simulink model "HybridInverter"  (R2024b)
settings: Solver=ode23t  StartTime=0.0  StopTime=1  RelTol=1e-3
undefined symbols (not defined in the file): Ion, Lithium
libraries: spsCurrentMeasurementLib x8, spsSeriesRLCBranchLib x8, spsVoltageMeasurementLib x8, spsIGBTDiodeLib x7, spsIdealSwitchLib x5, slpidlib x3, spsSeriesRLCLoadLib x3, spsFirstOrderFilterLib x2, simulink x2, spsACVoltageSourceLib x1, spsAlphaBetaZerotodq0Lib x1, spsBatteryLib x1
settings Model: SimulationMode=accelerator  Creator=USER  LastModifiedBy=USER

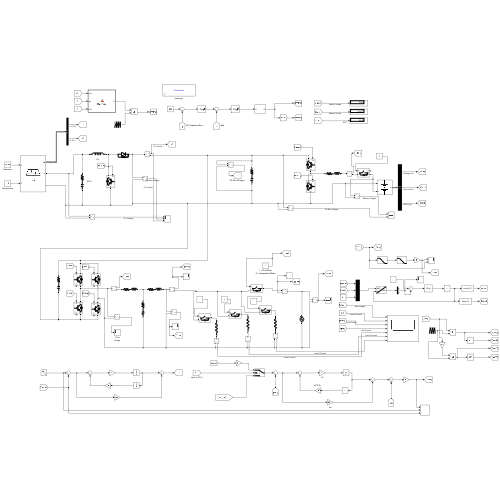
[thumbnail: Simulink's stored preview of the top-level diagram]
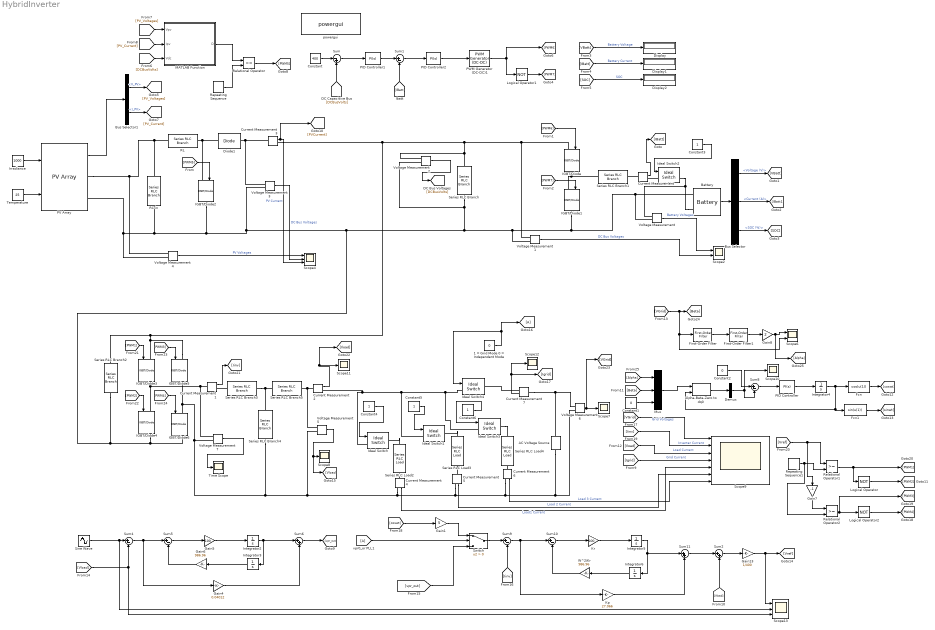
== system HybridInverter ==
  1 = Grid Mode 0 = Independent Mode : Constant  Value=0
  AC Voltage Source : spsACVoltageSourceLib/AC Voltage Source  Amplitude=325  Phase=0  Frequency=50  SampleTime=0  Measurements=None  BusType=swing  Pref=10e3  Qref=0  Qmin=-inf  Qmax=+inf
  Alpha-Beta-Zero to dq0 : spsAlphaBetaZerotodq0Lib/Alpha-Beta-Zero to dq0  Alignment=90 degrees behind phase A axis
  Battery : spsBatteryLib/Battery  BatType=Lithium-Ion  NomV=200  NomQ=15  SOC=55  Batt_Tr=1  PresetModel=on  MaxQ=15  MinV=150  FullV=232.7974  Dis_rate=6.5217  R=0.13333  Normal_OP=13.5652  expZone="[216.0772     0.7369565]"
  Bus Selector : BusSelector  OutputSignals=Voltage (V),Current (A),SOC (%)
  Bus Selector1 : BusSelector  OutputSignals=V_PV,I_PV
  Constant : Constant  Value=400
  Constant1 : Constant  Value=0
  Constant2 : Constant  Value=0
  Constant{3..6} (4 alike) : Constant
  Current Measurement{,1..7} (8 alike) : spsCurrentMeasurementLib/Current Measurement  PhasorSimulation=off  OutputType=Complex  PSBequivalent=0
  Demux : Demux  Outputs=3
  Diode1 : spsDiodeLib/Diode  Ron=0.001  Lon=0  Vf=0.8  IC=0  UseSnubber=0  Rs=500  Cs=250e-9  Measurements=off
  Display : Display
  Display1 : Display
  Display2 : Display
  Fcn : Fcn  Expr=cos(u(1))
  Fcn1 : Fcn  Expr=sin(u(1))
  First-Order Filter : spsFirstOrderFilterLib/First-Order Filter  FilterType=Lowpass  Tc=1/(2*pi*50)  Ts=0  Initialize=off  Vac_Init=[0, 0, 60]  Vdc_Init=0  PlotResponse=off  FreqRange="[0,  200,  1]"
  First-Order Filter1 : spsFirstOrderFilterLib/First-Order Filter  FilterType=Lowpass  Tc=1/(2*pi*50)  Ts=0  Initialize=off  Vac_Init=[0, 0, 60]  Vdc_Init=0  PlotResponse=off  FreqRange="[0,  200,  1]"
  Gain1 : Gain  Gain=5
  Gain13 : Gain  Gain=1/400
  Gain4 : Gain  Gain=0.04012
  Gain5 : Gain  Gain=100
  Gain6 : Gain  Gain=986.96
  Gain7 : Gain  Gain=-1
  Gain8 : Gain  Gain=2
  Goto16 : Goto
  IGBT/Diode : spsIGBTDiodeLib/IGBT//Diode  Ron=1e-3  Rs=1e5  Cs=inf  Measurements=off
  IGBT/Diode1 : spsIGBTDiodeLib/IGBT//Diode  Ron=1e-3  Rs=1e5  Cs=inf  Measurements=off
  IGBT/Diode2 : spsIGBTDiodeLib/IGBT//Diode  Ron=1e-3  Rs=1e5  Cs=inf  Measurements=off
  IGBT/Diode{3..6} (4 alike) : spsIGBTDiodeLib/IGBT//Diode  Ron=1e-3  Rs=1e5  Cs=inf  Measurements=on
  Ideal Switch{,1,3..4} (4 alike) : spsIdealSwitchLib/Ideal Switch  Ron=0.001  Lon=0  IC=0  Rs=1e5  Cs=inf  Measurements=off
  Ideal Switch2 : spsIdealSwitchLib/Ideal Switch  Ron=0.001  Lon=0  IC=0  Rs=1e5  Cs=inf  Measurements=on
  Integrator{2..6} (5 alike) : Integrator
  Irradiance : Constant  Value=1000
  Kp : Gain  Gain=27.066
  Kr : Gain  Gain=100
  Logical Operator : Logic  Operator=NOT  AllPortsSameDT=off  OutDataTypeStr=boolean
  Logical Operator1 : Logic  Operator=NOT  AllPortsSameDT=off  OutDataTypeStr=boolean
  Logical Operator2 : Logic  Operator=NOT  AllPortsSameDT=off  OutDataTypeStr=boolean
  MATLAB Function : MATLAB Function  TreatAsAtomicUnit=on
  Mux : Mux  Inputs=3
  PID Controller : slpidlib/PID Controller  Controller=PI  Form=Parallel  TimeDomain=Continuous-time  UseExternalTs=off  SampleTime=-1  IntegratorMethod=Forward Euler  FilterMethod=Forward Euler  ControllerParametersSource=internal  P=10  I=50000  UseKiTs=off  D=0  UseExternalDerivativeSource=off  N=100  UseFilter=on  TunerSelectOption=Transfer Function Based (PID Tuner App)  InitialConditionSource=internal  InitialConditionForIntegrator=0  InitialConditionForFilter=0  DifferentiatorICPrevScaledInput=0  ExternalReset=none  TrackingMode=off  Kt=1  LimitOutput=off  SatLimitsSource=internal  UpperSaturationLimit=inf  LowerSaturationLimit=-inf  LinearizeAsGain=on  AntiWindupMode=none  Kb=1  LimitIntegrator=off  UpperIntegratorSaturationLimit=inf  LowerIntegratorSaturationLimit=-inf  POutMin=[]  POutMax=[]  IOutMin=[]  IOutMax=[]  DOutMin=[]  DOutMax=[]  NOutMin=[]  NOutMax=[]  SumOutMin=[]  SumOutMax=[]  SaturationOutMin=[]  SaturationOutMax=[]  PParamMin=[]  PParamMax=[]  IParamMin=[]  IParamMax=[]  DParamMin=[]  DParamMax=[]  NParamMin=[]  NParamMax=[]  KbParamMin=[]  KbParamMax=[]  KtParamMin=[]  KtParamMax=[]  KbOutMin=[]  KbOutMax=[]  KtOutMin=[]  KtOutMax=[]  IntegratorOutMin=[]  IntegratorOutMax=[]  FilterOutMin=[]  FilterOutMax=[]  SumI1OutMin=[]  SumI1OutMax=[]  SumI2OutMin=[]  SumI2OutMax=[]  SumI3OutMin=[]  SumI3OutMax=[]  SumI4OutMin=[]  SumI4OutMax=[]  SumDOutMin=[]  SumDOutMax=[]  DifferentiatorOutMin=[]  DifferentiatorOutMax=[]  FilterDiffOutCoefMin=[]  FilterDiffOutCoefMax=[]  ReciprocalOutMin=[]  ReciprocalOutMax=[]  SumDenOutMin=[]  SumDenOutMax=[]  SumNumOutMin=[]  SumNumOutMax=[]  DivideOutMin=[]  DivideOutMax=[]  UdiffTsProdOutMin=[]  UdiffTsProdOutMax=[]  NTsProdOutMin=[]  NTsProdOutMax=[]  UintegralTsProdOutMin=[]  UintegralTsProdOutMax=[]  UngainTsProdOutMin=[]  UngainTsProdOutMax=[]  ClampingZeroOutDataTypeStr=Inherit: Inherit via back propagation  ClampingZeroOutMin=[]  ClampingZeroOutMax=[]  FilterDenConstantOutDataTypeStr=Inherit: Inherit via back propagation  FilterDenConstantOutMin=[]  FilterDenConstantOutMax=[]  PCopyOutDataTypeStr=Inherit: Inherit via back propagation  PCopyOutMin=[]  PCopyOutMax=[]  NCopyOutDataTypeStr=Inherit: Inherit via back propagation  NCopyOutMin=[]  NCopyOutMax=[]  IntegratorContinuousStateAttributes=''  IntegratorStateMustResolveToSignalObject=off  IntegratorRTWStateStorageClass=Auto  FilterContinuousStateAttributes=''  FilterStateMustResolveToSignalObject=off  FilterRTWStateStorageClass=Auto  ParallelPVariant=InternalParameters  IdealPVariant=Disabled  IVariant=InternalParameters  DVariant=Disabled  IntegratorVariant=Continuous  SatVariant=Disabled  AWVariant=Passthrough  PCopyVariant=Disabled  TRVariant=Disabled  FdbkBlocksVariant=Forward  IdealPFdbkVariant=Disabled  SatFdbkVariant=Disabled  DerivativeFilterVariant=Disabled  NVariant=Disabled  NCopyVariant=Disabled_SignalSpec  FilterICVariant=Disabled  IntegratorICVariant=InternalICs  ExternalResetVariant=Disabled  TRSumVariant=Passthrough  SumFdbkVariant=Disabled  SumVariant=Sum_PI  TsampFilterVariant=InternalTs  TsampNgainVariant=Passthrough  TsampIntegralVariant=Disabled_SignalSpec  ExternalSaturationOutDataTypeStr=Inherit: Same as second input  DerivativeSourceVariant=Disabled  PreIntVariant=InternalPreInt
  PID Controller1 : slpidlib/PID Controller  Controller=PI  Form=Parallel  TimeDomain=Continuous-time  UseExternalTs=off  SampleTime=-1  IntegratorMethod=Forward Euler  FilterMethod=Forward Euler  ControllerParametersSource=internal  P=5  I=2  UseKiTs=off  D=0  UseExternalDerivativeSource=off  N=100  UseFilter=on  TunerSelectOption=Transfer Function Based (PID Tuner App)  ZeroCross=off  InitialConditionSource=internal  InitialConditionForIntegrator=0  InitialConditionForFilter=0  DifferentiatorICPrevScaledInput=0  ExternalReset=none  TrackingMode=off  Kt=1  LimitOutput=on  SatLimitsSource=internal  UpperSaturationLimit=15  LowerSaturationLimit=-15  LinearizeAsGain=on  AntiWindupMode=none  Kb=1  LimitIntegrator=off  UpperIntegratorSaturationLimit=inf  LowerIntegratorSaturationLimit=-inf  POutMin=[]  POutMax=[]  IOutMin=[]  IOutMax=[]  DOutMin=[]  DOutMax=[]  NOutMin=[]  NOutMax=[]  SumOutMin=[]  SumOutMax=[]  SaturationOutMin=[]  SaturationOutMax=[]  PParamMin=[]  PParamMax=[]  IParamMin=[]  IParamMax=[]  DParamMin=[]  DParamMax=[]  NParamMin=[]  NParamMax=[]  KbParamMin=[]  KbParamMax=[]  KtParamMin=[]  KtParamMax=[]  KbOutMin=[]  KbOutMax=[]  KtOutMin=[]  KtOutMax=[]  IntegratorOutMin=[]  IntegratorOutMax=[]  FilterOutMin=[]  FilterOutMax=[]  SumI1OutMin=[]  SumI1OutMax=[]  SumI2OutMin=[]  SumI2OutMax=[]  SumI3OutMin=[]  SumI3OutMax=[]  SumI4OutMin=[]  SumI4OutMax=[]  SumDOutMin=[]  SumDOutMax=[]  DifferentiatorOutMin=[]  DifferentiatorOutMax=[]  FilterDiffOutCoefMin=[]  FilterDiffOutCoefMax=[]  ReciprocalOutMin=[]  ReciprocalOutMax=[]  SumDenOutMin=[]  SumDenOutMax=[]  SumNumOutMin=[]  SumNumOutMax=[]  DivideOutMin=[]  DivideOutMax=[]  UdiffTsProdOutMin=[]  UdiffTsProdOutMax=[]  NTsProdOutMin=[]  NTsProdOutMax=[]  UintegralTsProdOutMin=[]  UintegralTsProdOutMax=[]  UngainTsProdOutMin=[]  UngainTsProdOutMax=[]  ClampingZeroOutDataTypeStr=Inherit: Inherit via back propagation  ClampingZeroOutMin=[]  ClampingZeroOutMax=[]  FilterDenConstantOutDataTypeStr=Inherit: Inherit via back propagation  FilterDenConstantOutMin=[]  FilterDenConstantOutMax=[]  PCopyOutDataTypeStr=Inherit: Inherit via back propagation  PCopyOutMin=[]  PCopyOutMax=[]  NCopyOutDataTypeStr=Inherit: Inherit via back propagation  NCopyOutMin=[]  NCopyOutMax=[]  IntegratorContinuousStateAttributes=''  IntegratorStateMustResolveToSignalObject=off  IntegratorRTWStateStorageClass=Auto  FilterContinuousStateAttributes=''  FilterStateMustResolveToSignalObject=off  FilterRTWStateStorageClass=Auto  ParallelPVariant=InternalParameters  IdealPVariant=Disabled  IVariant=InternalParameters  DVariant=Disabled  IntegratorVariant=Continuous  SatVariant=Enabled  AWVariant=Passthrough  PCopyVariant=Disabled  TRVariant=Disabled  FdbkBlocksVariant=Forward  IdealPFdbkVariant=Disabled  SatFdbkVariant=Disabled  DerivativeFilterVariant=Disabled  NVariant=Disabled  NCopyVariant=Disabled_SignalSpec  FilterICVariant=Disabled  IntegratorICVariant=InternalICs  ExternalResetVariant=Disabled  TRSumVariant=Passthrough  SumFdbkVariant=Disabled  SumVariant=Sum_PI  TsampFilterVariant=InternalTs  TsampNgainVariant=Passthrough  TsampIntegralVariant=Disabled_SignalSpec  ExternalSaturationOutDataTypeStr=Inherit: Same as second input  DerivativeSourceVariant=Disabled  PreIntVariant=InternalPreInt
  PID Controller2 : slpidlib/PID Controller  Controller=PI  Form=Parallel  TimeDomain=Continuous-time  UseExternalTs=off  SampleTime=-1  IntegratorMethod=Forward Euler  FilterMethod=Forward Euler  ControllerParametersSource=internal  P=0.2  I=200  UseKiTs=off  D=0  UseExternalDerivativeSource=off  N=100  UseFilter=on  TunerSelectOption=Transfer Function Based (PID Tuner App)  ZeroCross=off  InitialConditionSource=internal  InitialConditionForIntegrator=0  InitialConditionForFilter=0  DifferentiatorICPrevScaledInput=0  ExternalReset=none  TrackingMode=off  Kt=1  LimitOutput=on  SatLimitsSource=internal  UpperSaturationLimit=0.95  LowerSaturationLimit=0  LinearizeAsGain=on  AntiWindupMode=none  Kb=1  LimitIntegrator=off  UpperIntegratorSaturationLimit=inf  LowerIntegratorSaturationLimit=-inf  POutMin=[]  POutMax=[]  IOutMin=[]  IOutMax=[]  DOutMin=[]  DOutMax=[]  NOutMin=[]  NOutMax=[]  SumOutMin=[]  SumOutMax=[]  SaturationOutMin=[]  SaturationOutMax=[]  PParamMin=[]  PParamMax=[]  IParamMin=[]  IParamMax=[]  DParamMin=[]  DParamMax=[]  NParamMin=[]  NParamMax=[]  KbParamMin=[]  KbParamMax=[]  KtParamMin=[]  KtParamMax=[]  KbOutMin=[]  KbOutMax=[]  KtOutMin=[]  KtOutMax=[]  IntegratorOutMin=[]  IntegratorOutMax=[]  FilterOutMin=[]  FilterOutMax=[]  SumI1OutMin=[]  SumI1OutMax=[]  SumI2OutMin=[]  SumI2OutMax=[]  SumI3OutMin=[]  SumI3OutMax=[]  SumI4OutMin=[]  SumI4OutMax=[]  SumDOutMin=[]  SumDOutMax=[]  DifferentiatorOutMin=[]  DifferentiatorOutMax=[]  FilterDiffOutCoefMin=[]  FilterDiffOutCoefMax=[]  ReciprocalOutMin=[]  ReciprocalOutMax=[]  SumDenOutMin=[]  SumDenOutMax=[]  SumNumOutMin=[]  SumNumOutMax=[]  DivideOutMin=[]  DivideOutMax=[]  UdiffTsProdOutMin=[]  UdiffTsProdOutMax=[]  NTsProdOutMin=[]  NTsProdOutMax=[]  UintegralTsProdOutMin=[]  UintegralTsProdOutMax=[]  UngainTsProdOutMin=[]  UngainTsProdOutMax=[]  ClampingZeroOutDataTypeStr=Inherit: Inherit via back propagation  ClampingZeroOutMin=[]  ClampingZeroOutMax=[]  FilterDenConstantOutDataTypeStr=Inherit: Inherit via back propagation  FilterDenConstantOutMin=[]  FilterDenConstantOutMax=[]  PCopyOutDataTypeStr=Inherit: Inherit via back propagation  PCopyOutMin=[]  PCopyOutMax=[]  NCopyOutDataTypeStr=Inherit: Inherit via back propagation  NCopyOutMin=[]  NCopyOutMax=[]  IntegratorContinuousStateAttributes=''  IntegratorStateMustResolveToSignalObject=off  IntegratorRTWStateStorageClass=Auto  FilterContinuousStateAttributes=''  FilterStateMustResolveToSignalObject=off  FilterRTWStateStorageClass=Auto  ParallelPVariant=InternalParameters  IdealPVariant=Disabled  IVariant=InternalParameters  DVariant=Disabled  IntegratorVariant=Continuous  SatVariant=Enabled  AWVariant=Passthrough  PCopyVariant=Disabled  TRVariant=Disabled  FdbkBlocksVariant=Forward  IdealPFdbkVariant=Disabled  SatFdbkVariant=Disabled  DerivativeFilterVariant=Disabled  NVariant=Disabled  NCopyVariant=Disabled_SignalSpec  FilterICVariant=Disabled  IntegratorICVariant=InternalICs  ExternalResetVariant=Disabled  TRSumVariant=Passthrough  SumFdbkVariant=Disabled  SumVariant=Sum_PI  TsampFilterVariant=InternalTs  TsampNgainVariant=Passthrough  TsampIntegralVariant=Disabled_SignalSpec  ExternalSaturationOutDataTypeStr=Inherit: Same as second input  DerivativeSourceVariant=Disabled  PreIntVariant=InternalPreInt
  PV Array : spsPVArrayLib/PV Array  Npar=2  Nser=6  PlotType=array @ 1000 W/m2 & specified temperatures  S_vec="[ 1000  500  100 ]"  Temp_C_vec="[ 45 25  ]"  ModuleName=User-defined  PlotWhenSelected=off  Pm=213.15  Ncell=60  Voc=36.3  Isc=7.48  Vm=29  Im=7.35  beta_Voc_pc=-0.36099  alpha_Isc_pc=0.102  beta_Voc=-0.13104  alpha_Isc=0.0076296  IL=7.6859  I0=2.8063e-10  nI=0.97986  Rsh=3440.9004  Rs=0.39873  RobustModel=off  RobustCellTemperature=313.3991  BAL=on  Tc=1e-6  Tfilter=5e-5
  PWM Generator (DC-DC)1 : spsPWMGeneratorDCDCLib/PWM Generator (DC-DC)  Fsw=20000  Ts=1e-6
  RC in : spsSeriesRLCBranchLib/Series RLC Branch  LConnTagsString=__new0  RConnTagsString=__new0  BranchType=RC  Resistance=10e-4  Inductance=1e-3  SetiL0=off  InitialCurrent=0  Capacitance=100e-7  Setx0=off  InitialVoltage=0  Measurements=None
  RL : spsSeriesRLCBranchLib/Series RLC Branch  LConnTagsString=__new0  RConnTagsString=__new0  BranchType=L  Resistance=0  Inductance=1.45e-3  SetiL0=off  InitialCurrent=0  Capacitance=1e-6  Setx0=off  InitialVoltage=0  Measurements=None
  Relational Operator : RelationalOperator  OutDataTypeStr=boolean  RndMeth=Simplest  InputSameDT=off
  Relational Operator1 : RelationalOperator  OutDataTypeStr=boolean  RndMeth=Simplest  InputSameDT=off
  Relational Operator2 : RelationalOperator  OutDataTypeStr=boolean  RndMeth=Simplest  InputSameDT=off
  Repeating Sequence : simulink/Sources/Repeating Sequence  rep_seq_t=[0 0.00005]  rep_seq_y=[0 1]
  Repeating Sequence1 : simulink/Sources/Repeating Sequence  rep_seq_t=[0 0.00005 0.0001]  rep_seq_y=[-1 1 -1]
  Scope{7..8,10..12} (5 alike) : Scope
  Scope13 : Scope  NumInputPorts=3
  Scope2 : Scope  NumInputPorts=2
  Scope4 : Scope  NumInputPorts=3
  Scope6 : Scope  NumInputPorts=2
  Scope9 : Scope  NumInputPorts=7
  Series RLC Branch : spsSeriesRLCBranchLib/Series RLC Branch  LConnTagsString=__new0  RConnTagsString=__new0  BranchType=RC  Resistance=1e-4  Inductance=1e-3  SetiL0=off  InitialCurrent=0  Capacitance=3120e-6  Setx0=on  InitialVoltage=385  Measurements=None
  Series RLC Branch1 : spsSeriesRLCBranchLib/Series RLC Branch  LConnTagsString=__new0  RConnTagsString=__new0  BranchType=RL  Resistance=0.1  Inductance=1e-3  SetiL0=off  InitialCurrent=0  Capacitance=13e-3  Setx0=off  InitialVoltage=0  Measurements=None
  Series RLC Branch2 : spsSeriesRLCBranchLib/Series RLC Branch  LConnTagsString=__new0  RConnTagsString=__new0  BranchType=RC  Resistance=0.0042  Inductance=1e-3  SetiL0=off  InitialCurrent=0  Capacitance=500e-6  Setx0=off  InitialVoltage=0  Measurements=None
  Series RLC Branch3 : spsSeriesRLCBranchLib/Series RLC Branch  LConnTagsString=__new0  RConnTagsString=__new0  BranchType=RL  Resistance=0.001  Inductance=4.06e-3  SetiL0=off  InitialCurrent=0  Capacitance=1e-6  Setx0=off  InitialVoltage=0  Measurements=None
  Series RLC Branch4 : spsSeriesRLCBranchLib/Series RLC Branch  LConnTagsString=__new0  RConnTagsString=__new0  BranchType=RC  Resistance=0.0042  Inductance=1e-3  SetiL0=off  InitialCurrent=0  Capacitance=6.0175e-6  Setx0=off  InitialVoltage=0  Measurements=None
  Series RLC Branch5 : spsSeriesRLCBranchLib/Series RLC Branch  LConnTagsString=__new0  RConnTagsString=__new0  BranchType=RL  Resistance=0.001  Inductance=4.35e-3  SetiL0=off  InitialCurrent=0  Capacitance=1e-6  Setx0=off  InitialVoltage=0  Measurements=None
  Series RLC Load2 : spsSeriesRLCLoadLib/Series RLC Load  LConnTagsString=a  RConnTagsString=__new0  NominalVoltage=230  NominalFrequency=50  ActivePower=75  InductivePower=0  CapacitivePower=0  Setx0=off  InitialVoltage=0  SetiL0=off  InitialCurrent=0  Measurements=None  LoadType=constant Z
  Series RLC Load3 : spsSeriesRLCLoadLib/Series RLC Load  LConnTagsString=a  RConnTagsString=__new0  NominalVoltage=230  NominalFrequency=50  ActivePower=80  InductivePower=0  CapacitivePower=0  Setx0=off  InitialVoltage=0  SetiL0=off  InitialCurrent=0  Measurements=None  LoadType=constant Z
  Series RLC Load4 : spsSeriesRLCLoadLib/Series RLC Load  LConnTagsString=a  RConnTagsString=__new0  NominalVoltage=230  NominalFrequency=50  ActivePower=50  InductivePower=0  CapacitivePower=0  Setx0=off  InitialVoltage=0  SetiL0=off  InitialCurrent=0  Measurements=None  LoadType=constant Z
  Sine Wave : Sin  Amplitude=230  Frequency=314.16  SampleTime=0
  Sum : Sum  Inputs=|-+
  Sum{1,4..5,8..10} (6 alike) : Sum  Inputs=|+-
  Sum11 : Sum  Inputs=|++
  Sum2 : Sum  Inputs=|++
  Sum6 : Sum  Inputs=|++
  Switch : Switch  Criteria=u2 > Threshold  SaturateOnIntegerOverflow=off  InputSameDT=off
  Temperature : Constant  Value=25
  Time Scope : Scope
  Voltage Measurement{,1..7} (8 alike) : spsVoltageMeasurementLib/Voltage Measurement  PhasorSimulation=off  OutputType=Complex  PSBequivalent=0
  W^2/Kr : Gain  Gain=986.96
  powergui : sps_lib/powergui  Priority=1  SimulationMode=Continuous  SampleTime=1e-6  frequency=60  Iterations=50  frequencyindice=0  Pbase=100e6  ErrMax=1e-4  UnitsV=kV  UnitsW=MW  buscounter=0  FunctionMessages=off  echomessages=off  EnableUseOfTLC=off  CurrentSourceSwitches=off  DisableSnubberDevices=off  DisableRonSwitches=off  DisableVfSwitches=off  DisplayEquations=off  AutomaticDiscreteSolvers=off  SolverType=Tustin/Backward Euler (TBE)  Interpol=off  ExternalGateDelay=off  methode=off  Ts=100  x0status=blocks  SPID=on  SwTol=0  HookPort=off  NonlinearTolerance=1e-4  nMaxIteration=100  ContinueOnMaxIteration=off  RestoreLinks=warning  ResistiveCurrentMeasurement=off  Frange=[0:2:500]  Ylog=off  Xlog=on  ShowGrid=off  save=off  variable=ZData  structure=0  ZoomFFT=off  StartTime=0.0  cycles=1  DisplayStyle=1  fundamental=60  FreqAxis=off  MaxFrequency=1000  frequencyindicesteady=1  RmsSteady=1  display=off
  vpr0_or PLL1 : From
  wires:
  [IBatt] -> Display1/1  "Battery Current"
  [PWM5] -> IGBT/Diode2/1
  [SOC] -> Display2/1  "SOC"
  [PWM7] -> IGBT/Diode1/1
  Bus Selector/2 -> [IBatt1]  "<Current (A)>"
  PV Array/1 -> Bus Selector1/1
  [IBatt] -> Sum1/2
  [DCBusVolts] -> MATLAB Function/3(Vdc)
  Voltage Measurement3/1 -> Scope4/2  "DC Bus Voltages"
  Repeating Sequence/1 -> Relational Operator/2
  MATLAB Function/1(D) -> Relational Operator/1
  PID Controller2/1 -> PWM Generator (DC-DC)1/1
  Bus Selector1/2 -> [PV_Current]  "<I_PV>"
  Bus Selector/1 -> [VBatt]  "<Voltage (V)>"
  Sum1/1 -> PID Controller2/1
  Current Measurement3/1 -> [PVCurrent], Scope4/3  "PV Current"
  Temperature/1 -> PV Array/2
  PID Controller1/1 -> Sum1/1
  Relational Operator/1 -> [PWM5]
  [DCBusVolts] -> Sum/2
  [PV_Voltages] -> MATLAB Function/1(Vpv)
  Constant3/1 -> Ideal Switch2/1
  PWM Generator (DC-DC)1/1 -> [PWM6], Logical Operator1/1
  Constant/1 -> Sum/1
  [PWM6] -> IGBT/Diode/1
  Sum/1 -> PID Controller1/1
  Current Measurement/1 -> [IBatt]
  Voltage Measurement1/1 -> Scope2/2  "DC Bus Voltages"
  Irradiance/1 -> PV Array/1
  Logical Operator1/1 -> [PWM7]
  Bus Selector1/1 -> [PV_Voltages]  "<V_PV>"
  Battery/1 -> Bus Selector/1
  [VBatt] -> Display/1  "Battery Voltage"
  [PV_Current] -> MATLAB Function/2(Ipv)
  Voltage Measurement/1 -> Scope2/1  "Battery Voltages"
  Voltage Measurement2/1 -> [DCBusVolts]
  Voltage Measurement4/1 -> Scope4/1  "PV Voltages"
  Bus Selector/3 -> [SOC]  "<SOC (%)>"
  Logical Operator/1 -> [PWM2]
  Switch/1 -> Sum9/1
  Kr/1 -> Integrator5/1
  Mux/1 -> Alpha-Beta-Zero to dq0/1
  Voltage Measurement7/1 -> Time Scope/1
  Constant2/1 -> Sum8/1
  [Beta] -> Mux/2
  [PWM3] -> IGBT/Diode5/1
  Current Measurement6/1 -> Scope9/7  "Load 3 Current"
  Gain1/1 -> Switch/1
  Constant4/1 -> Ideal Switch/1
  Gain8/1 -> [Alpha], Scope6/1
  Demux/2 -> Scope10/1, Sum8/2
  [Vload] -> Sum4/2, Scope13/3
  [Iinv] -> Scope9/2  "Inverter Current"
  First-Order Filter/1 -> First-Order Filter1/1
  [coswt] -> Gain1/1
  Voltage Measurement6/1 -> [VGrid], Scope7/1
  Fcn/1 -> [coswt]
  Integrator6/1 -> W^2/Kr/1
  Constant5/1 -> Ideal Switch1/1
  Sum8/1 -> PID Controller/1
  Relational Operator1/1 -> [PWM1], Logical Operator/1
  [Iload] -> Scope9/3  "Load Current"
  PID Controller/1 -> Integrator4/1
  Fcn1/1 -> [sinwt]
  Sine Wave/1 -> Scope13/2, Sum4/1
  Current Measurement1/1 -> [Iinv]
  [Iinv] -> Sum9/2
  Current Measurement5/1 -> Scope9/6  "Load 2 Current"
  [Vload] -> Sum2/2
  Gain6/1 -> Sum5/2
  Sum4/1 -> Gain4/1, Sum5/1
  [Vref] -> Gain7/1, Relational Operator1/1
  Sum11/1 -> Sum2/1
  [VGrid] -> [Beta], Scope6/2, First-Order Filter/1
  Constant1/1 -> Mux/3
  Integrator4/1 -> Alpha-Beta-Zero to dq0/2, Fcn1/1, Fcn/1
  vpr0_or PLL1/1 -> Switch/2
  Gain13/1 -> [Vref], Scope13/1
  Sum2/1 -> Gain13/1
  Sum5/1 -> Gain5/1
  Repeating Sequence1/1 -> Relational Operator2/2, Relational Operator1/2
  Integrator5/1 -> Integrator6/1, Sum11/1
  Sum9/1 -> Kp/1, Sum10/1
  Current Measurement2/1 -> [Iload], Scope11/1
  W^2/Kr/1 -> Sum10/2
  [PWM1] -> IGBT/Diode3/1
  Sum6/1 -> [vpr_out]
  Voltage Measurement5/1 -> [Vload], Scope8/1
  [VGrid] -> Scope9/1  "Grid Voltages"
  Current Measurement7/1 -> [Igrid], Scope12/1
  Current Measurement4/1 -> Scope9/5  "Load1 Current"
  [Igrid] -> Scope9/4  "Grid Current"
  Logical Operator2/1 -> [PWM4]
  Integrator3/1 -> Gain6/1
  Gain4/1 -> Sum6/2
  [Alpha] -> Mux/1
  Integrator2/1 -> Sum6/1, Integrator3/1
  First-Order Filter1/1 -> Gain8/1
  Constant6/1 -> Ideal Switch3/1
  [vpr_out] -> Switch/3
  Gain5/1 -> Integrator2/1
  [PWM4] -> IGBT/Diode6/1
  Gain7/1 -> Relational Operator2/1
  Kp/1 -> Sum11/2
  Sum10/1 -> Kr/1
  [PWM2] -> IGBT/Diode4/1
  1 = Grid Mode 0 = Independent Mode/1 -> Goto16/1, Ideal Switch4/1
  Relational Operator2/1 -> [PWM3], Logical Operator2/1
  Alpha-Beta-Zero to dq0/1 -> Demux/1
  connections:
  IGBT/Diode5/LConn1 -- IGBT/Diode3/LConn1 -- Series RLC Branch2/LConn1 -- Voltage Measurement1/LConn1 -- IGBT/Diode/LConn1 -- Series RLC Branch/LConn1 -- Voltage Measurement2/LConn1 -- Current Measurement3/RConn1
  IGBT/Diode1/LConn1 -- IGBT/Diode/RConn1 -- Series RLC Branch1/LConn1
  PV Array/RConn1 -- RL/LConn1 -- RC in/LConn1 -- Voltage Measurement4/LConn1
  Diode1/LConn1 -- RL/RConn1 -- IGBT/Diode2/LConn1
  IGBT/Diode4/RConn1 -- Series RLC Branch2/RConn1 -- Voltage Measurement1/LConn2 -- Voltage Measurement/LConn2 -- Battery/LConn2 -- IGBT/Diode1/RConn1 -- Series RLC Branch/RConn1 -- Voltage Measurement2/LConn2 -- IGBT/Diode2/RConn1 -- Voltage Measurement4/LConn2 -- PV Array/RConn2 -- RC in/RConn1 -- Voltage Measurement3/LConn2 -- IGBT/Diode6/RConn1
  Battery/LConn1 -- Voltage Measurement/LConn1 -- Ideal Switch2/RConn1
  Diode1/RConn1 -- Voltage Measurement3/LConn1 -- Current Measurement3/LConn1
  Ideal Switch2/LConn1 -- Current Measurement/RConn1
  Current Measurement/LConn1 -- Series RLC Branch1/RConn1
  Series RLC Branch5/RConn1 -- Current Measurement2/LConn1 -- Voltage Measurement5/LConn1
  IGBT/Diode3/RConn1 -- Voltage Measurement7/LConn1 -- Current Measurement1/LConn1 -- IGBT/Diode4/LConn1
  Series RLC Branch5/LConn1 -- Series RLC Branch4/LConn1 -- Series RLC Branch3/RConn1
  Current Measurement5/RConn1 -- AC Voltage Source/LConn1 -- Voltage Measurement6/LConn2 -- Current Measurement6/RConn1 -- Current Measurement4/RConn1 -- Voltage Measurement5/LConn2 -- Series RLC Branch4/RConn1 -- IGBT/Diode5/RConn1 -- IGBT/Diode6/LConn1 -- Voltage Measurement7/LConn2
  Ideal Switch4/LConn1 -- Ideal Switch/LConn1 -- Current Measurement2/RConn1 -- Ideal Switch1/LConn1 -- Ideal Switch3/LConn1
  Voltage Measurement6/LConn1 -- AC Voltage Source/RConn1 -- Current Measurement7/LConn1
  Series RLC Load3/LConn1 -- Ideal Switch1/RConn1
  Current Measurement7/RConn1 -- Ideal Switch4/RConn1
  Series RLC Load2/LConn1 -- Ideal Switch/RConn1
  Current Measurement6/LConn1 -- Series RLC Load4/RConn1
  Series RLC Branch3/LConn1 -- Current Measurement1/RConn1
  Ideal Switch3/RConn1 -- Series RLC Load4/LConn1
  Current Measurement4/LConn1 -- Series RLC Load2/RConn1
  Current Measurement5/LConn1 -- Series RLC Load3/RConn1

== matlab function HybridInverter/MATLAB Function ==
  settings: updateMethod=DISCRETE
  data: Vpv input; D output; Ipv input; Vdc input
function D = DutyRatio(Vpv, Ipv, Vdc)

% MPPT + PI Controlled Boost Converter
% Restructured to directly regulate and protect the DC Bus Voltage

% INPUTS:
% Vpv  -> PV Array Voltage
% Ipv  -> PV Array Current
% Vdc  -> DC Bus Voltage
%
% OUTPUT:
% D    -> Duty Cycle for PWM

% SYSTEM SETTINGS
Vdc_ref   = 400;      % Desired DC Bus Voltage (V)

Vpv_max   = 300;      % Maximum PV Operating Voltage
Vpv_min   = 0;        % Minimum PV Operating Voltage

Vref_init = 250;      % Initial MPPT Voltage Reference
deltaVref = 2;        % Increased from 1 to 2 for faster tracking speed

Dmax = 0.95;          % Maximum Duty Cycle
Dmin = 0.05;          % Minimum Duty Cycle (Raised slightly for circuit stability)


% RETUNED PI CONTROLLER GAINS FOR DC BUS REGULATION
% (Adjusted to react to Vdc error instead of Vpv error)
Kp = 0.05;            
Ki = 0.002;           


% SPEED STRATEGY (OPTIMIZED WINDOWS)
N = 40;               % Decreased from 300 to react 7.5x faster to loads
M = 20;               % Decreased from 150 to keep a balanced averaging window


% PERSISTENT VARIABLES
persistent Vold Pold Vrefold Dold integral
persistent V_sum I_sum count_index Vref_current

if isempty(Vold)

    Vold     = 0;
    Pold     = 0;

    Vrefold  = Vref_init;

    Dold     = 0.50;

    integral = 0;
    
    count_index  = 1;
    V_sum        = 0;
    I_sum        = 0;
    Vref_current = Vref_init;

end

% Increment execution counter
count_index = count_index + 1;

% Accumulate data only during the last M samples
if count_index >= (N-M)
    V_sum = V_sum + Vpv;
    I_sum = I_sum + Ipv;
end

% --- STEP 1-4: MPPT GENERATES SOLAR VOLTAGE REFERENCE ---
if count_index == N
    
    V_avg = V_sum / M;
    I_avg = I_sum / M;
    
    P = V_avg * I_avg;

    dV = V_avg - Vold;
    dP = P     - Pold;

    % Perturb & Observe Logic
    if dP ~= 0
        if dP < 0
            if dV < 0
                Vref_current = Vrefold + deltaVref;
            else
                Vref_current = Vrefold - deltaVref;
            end
        else
            if dV < 0
                Vref_current = Vrefold - deltaVref;
            else
                Vref_current = Vrefold + deltaVref;
            end
        end
    else
        Vref_current = Vrefold;
    end

    % Bound the Solar Voltage Reference
    Vref_current = max(min(Vref_current, Vpv_max), Vpv_min);
    
    % Update MPPT memory
    Vold    = V_avg;
    Pold    = P;
    Vrefold = Vref_current;
    
    % Reset counters
    count_index = 1;
    V_sum = 0;
    I_sum = 0;
else
    Vref_current = Vrefold;
end


% --- NEW CONTINUOUS PI CONTROL LOGIC (WHY IT WORKS NOW) ---

% STEP 5: CALCULATE DC BUS ERROR (Crucial change!)
% If Vdc drops below Vdc_ref, error becomes POSITIVE
error = Vdc_ref - Vdc;


% STEP 6: CORRECTED STANDARD PI CONTROLLER FORMULA
% Removed the unstable "+ Dold" accumulation from the inside step
integral = integral + error;

% Anti-Windup Protection: Stops the integral from growing infinitely if saturated
if integral > 50;  integral = 50;  end
if integral < -50; integral = -50; end

D_calculated = (Kp * error) + (Ki * integral);


% STEP 7: SOLAR EXTRACTION LIMITER
% If the solar panel voltage drops too low (collapsing), we override the duty 
% cycle to prevent the system from short-circuiting the solar panel array.
if Vpv < (Vref_current - 10)
    D_calculated = D_calculated - 0.05; 
end


% STEP 8: DUTY CYCLE SATURATION & ASSIGNMENT
D = max(min(D_calculated, Dmax), Dmin);


% STEP 9: UPDATE MEMORY VARIABLES
Dold = D;

end
